simulink model "Tq_comb_timing"  (R2022b)
settings: Solver=daessc  StartTime=0.0  StopTime=5  RelTol=1e-3
InitFcn:
  | %% Tq_comb_timing.slx
  | % InitFcn
  | %
  | spring_stiffness = 1e10;
  | viscous_friction_coeff = 10;
  | current_limit = 12.5;
  | %
  | torque_start_t = 1;
  | torque_fin_val = -45;
  | %
  | inertia_start_t = 11.5;
  | inertia_init_val = 0.1;
  | inertia_fin_val  = 0.2;
  | %
  | M1_start_t = 0;
  | M2_start_t = 2;
  | M3_start_t = 3;
StopFcn:
  | disp(['spring_stiffness was       ' num2str(spring_stiffness)])
  | disp('')
  | disp(['viscous_friction_coeff was ' num2str(viscous_friction_coeff)])
  | disp('')
libraries: fl_lib x73, nesl_utility x42, ee_lib x12, sdl_lib x12, slpidlib x3, SignalEditorBlockLib x1
(part 2 of 2)

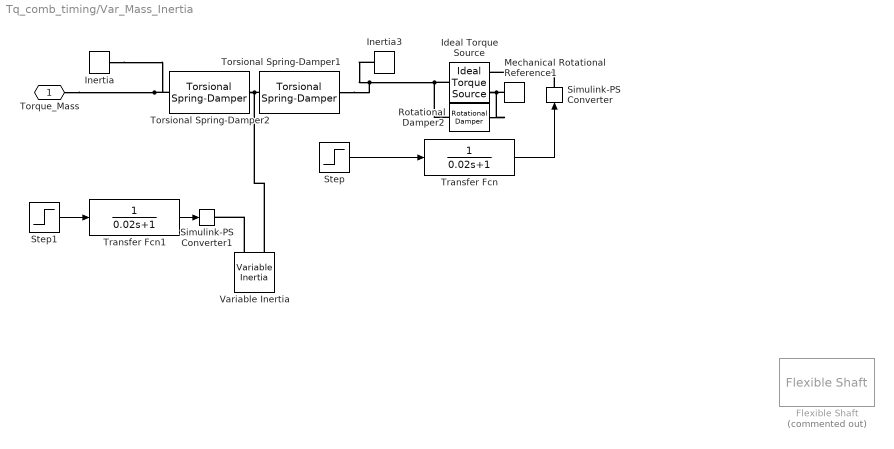
== system Tq_comb_timing/Var_Mass_Inertia ==
  Flexible Shaft : sdl_lib/Couplings & Drives/Flexible Shaft  Commented=on  modelTransverse=simscape.enum.onoff.off  n_segments=1  parameterization=sdl.enum.shaftParameterization.StiffnessInertia  length=1 m  lengths=[1, .5, .25] m  shaft_stiffness=2e5 N*m/rad  shaft_inertia=0.001 kg*m^2  shaft_stiffnesses=[400000, 200000, 100000] N*m/rad  shaft_inertias=[.025, .02, .015] kg*m^2  eiIN=5e5 Pa*m^4  rhoaIN=19 kg/m  eiINs=[600000, 500000, 400000] Pa*m^4  rhoaINs=[20, 19, 18] kg/m  density=7.8e3 kg/m^3  shear_modulus=7.93e9 Pa  elastic_modulus=200e9 Pa  shaft_construction=sdl.enum.shaftConstruction.solid  diameter_outer=0.075 m  diameter_inner=0.05 m  diameter_outers=[.085, .075, .065] m  diameter_inners=[.055, .05, .045] m  damping_ratio=0.01  mu_visc_BF=[0, 0] N*m*s/rad  mu_visc=[0, 0] N*m*s/rad  initial_deflection=0 rad  initial_velocity=0 rpm  num_supports=sdl.enum.num_supports.two  z_support=[0, 1] m  boundaryB1=sdl.enum.shaftSupport.clamp  DrotB1_row=[1000, 1000] N*m*s/rad  DtransB1_row=[20000, -44000, -44000, 350000] N*s/m  DtransB1_w_mat=[20000, -44000, -44000, 350000; 10000, -25000, -25000, 140000; 5000, -10000, -10000, 20000] N*s/m  KrotB1_row=[10000, 10000] N*m/rad  KtransB1_row=[1000000, -200000, -300000, 5000000] N/m  KtransB1_w_mat=[1000000, -600000, -3500000, 8000000; 1000000, -200000, -3000000, 5000000; 1000000, -50000, -2500000, 3000000] N/m  boundaryI1=sdl.enum.shaftSupport.clamp  DrotI1_row=[1000, 1000] N*m*s/rad  DtransI1_row=[20000, -44000, -44000, 350000] N*s/m  DtransI1_w_mat=[20000, -44000, -44000, 350000; 10000, -25000, -25000, 140000; 5000, -10000, -10000, 20000] N*s/m  KrotI1_row=[10000, 10000] N*m/rad  KtransI1_row=[1000000, -200000, -300000, 5000000] N/m  KtransI1_w_mat=[1000000, -600000, -3500000, 8000000; 1000000, -200000, -3000000, 5000000; 1000000, -50000, -2500000, 3000000] N/m  boundaryI2=sdl.enum.shaftSupport.clamp  DrotI2_row=[1000, 1000] N*m*s/rad  DtransI2_row=[20000, -44000, -44000, 350000] N*s/m  DtransI2_w_mat=[20000, -44000, -44000, 350000; 10000, -25000, -25000, 140000; 5000, -10000, -10000, 20000] N*s/m  KrotI2_row=[10000, 10000] N*m/rad  KtransI2_row=[1000000, -200000, -300000, 5000000] N/m  KtransI2_w_mat=[1000000, -600000, -3500000, 8000000; 1000000, -200000, -3000000, 5000000; 1000000, -50000, -2500000, 3000000] N/m  boundaryF1=sdl.enum.shaftSupport.clamp  DrotF1_row=[1000, 1000] N*m*s/rad  DtransF1_row=[20000, -44000, -44000, 350000] N*s/m  DtransF1_w_mat=[20000, -44000, -44000, 350000; 10000, -25000, -25000, 140000; 5000, -10000, -10000, 20000] N*s/m  KrotF1_row=[10000, 10000] N*m/rad  KtransF1_row=[1000000, -200000, -300000, 5000000] N/m  KtransF1_w_mat=[1000000, -600000, -3500000, 8000000; 1000000, -200000, -3000000, 5000000; 1000000, -50000, -2500000, 3000000] N/m  bearing_speed=[200, 500, 1500] rpm  alpha=10 1/s  beta=1e-8 s  noDisk=sdl.enum.shaftDisks.none  zDisk=0.5 m  mDiskIN=2 kg  IdDiskIN=0.025 kg*m^2  IpDiskIN=0.050 kg*m^2  offsetMR=[.01, .01] kg*m  offsetMassLocation=[.33, .67] m  offsetMR_initialAngleIN=[0, pi] rad  AnalysisMethod=sdl.enum.bendingAnalysisMethod.LumpedMass  ModeInputMethod=sdl.enum.modeInputMethod.SimscapeDetermined  numModesIn=6  mode_speed_dependency=sdl.enum.mode_speed_dependency.Static  OmegaNom=5000 rpm  wMax=1e8 rpm  dz=0.01 m  userMode_w=[280, 644, 615, 1285] rad/s  userMode_w_mat=[257, 780, 580, 1560; 280, 644, 615, 1285; 294, 513, 636, 1020] rad/s  userMode_z=[0, .1, .2, .3, .4, .5, .6, .7, .8, .9, 1] m  userMode_shapeX=[.1648, .0086, -.2759, .0162; .1671, .0093, -.2231, .0133; .1691, .01, -.1689, .0102; .1707, .0105, -.1135, .007; .1717, .0108, -.057, .0035; .1721, .0109, 0, 0; .1717, .0108, .057, -.0035; .1707, .0105, .1135, -.007; .1691, .01, .1689, -.0102; .1671, .0093, .2231, -.0133; .1648, .0086, .2759, -.0162]  userMode_shapeX_mat=cat(3, [.1842, .0134, -.3072, .0272; .1863, .0152, -.2482, .0226; .1882, .0169, -.1878, .0176; .1897, .0182, -.1261, .0121; .1906, .019, -.0634, .0062; .191, .0193, 0, 0; .1906, .019, .0634, -.0062; .1897, .0182, .1261, -.0121; .1882, .0169, .1878, -.0176; .1863, .0152, .2482, -.0226; .1842, .0134, .3072, -.0272], [.1648, .0086, -.2759, .0162; .1671, .0093, -.2231, .0133; .1691, .01, -.1689, .0102; .1707, .0105, -.1135, .007; .1717, .0108, -.057, .0035; .1721, .0109, 0, 0; .1717, .0108, .057, -.0035; .1707, .0105, .1135, -.007; .1691, .01, .1689, -.0102; .1671, .0093, .2231, -.0133; .1648, .0086, .2759, -.0162], [.1291, .0046, -.2166, .0082; .131, .0048, -.1751, .0067; .1327, .005, -.1327, .0051; .1341, .0052, -.0891, .0035; .135, .0053, -.0448, .0017; .1353, .0053, 0, 0; .135, .0053, .0448, -.0017; .1341, .0052, .0891, -.0035; .1327, .005, .1327, -.0051; .131, .0048, .1751, -.0067; .1291, .0046, .2166, -.0082])  userMode_shapeY=[.1193, -.1784, -.1997, -.3348; .1209, -.1933, -.1615, -.2751; .1224, -.2068, -.1223, -.2119; .1235, -.2176, -.0821, -.1445; .1243, -.2245, -.0413, -.0734; .1246, -.2269, 0, 0; .1243, -.2245, .0413, .0734; .1235, -.2176, .0821, .1445; .1224, -.2068, .1223, .2119; .1209, -.1933, .1615, .2751; .1193, -.1784, .1997, .3348]  userMode_shapeY_mat=cat(3, [.0885, -.1625, -.1475, -.3301; .0895, -.1847, -.1192, -.2745; .0904, -.2048, -.0902, -.2141; .0911, -.2209, -.0606, -.1475; .0916, -.2313, -.0304, -.0754; .0917, -.2349, 0, 0; .0916, -.2313, .0304, .0754; .0911, -.2209, .0606, .1475; .0904, -.2048, .0902, .2141; .0895, -.1847, .1192, .2745; .0885, -.1625, .1475, .3301], [.1193, -.1784, -.1997, -.3348; .1209, -.1933, -.1615, -.2751; .1224, -.2068, -.1223, -.2119; .1235, -.2176, -.0821, -.1445; .1243, -.2245, -.0413, -.0734; .1246, -.2269, 0, 0; .1243, -.2245, .0413, .0734; .1235, -.2176, .0821, .1445; .1224, -.2068, .1223, .2119; .1209, -.1933, .1615, .2751; .1193, -.1784, .1997, .3348], [.1566, -.1901, -.2628, -.3377; .1589, -.1994, -.2125, -.2753; .161, -.2079, -.1609, -.2103; .1627, -.2146, -.1081, -.1424; .1638, -.219, -.0544, -.0719; .1642, -.2205, 0, 0; .1638, -.219, .0544, .0719; .1627, -.2146, .1081, .1424; .161, -.2079, .1609, .2103; .1589, -.1994, .2125, .2753; .1566, -.1901, .2628, .3377])
      settings: InternalSimscapePortConfiguration="{\"Bottom\":[],\"Left\":[{\"id\":\"B\",\"label\":\"B\",\"type\":\"foundation.mechanical.rotational.rotational\"}],\"Right\":[{\"id\":\"F\",\"label\":\"F\",\"type\":\"foundation.mechanical.rotational.rotational\"}],\"Top\":[]}"
  Ideal Torque Source : fl_lib/Mechanical/Mechanical Sources/Ideal Torque Source
  Inertia : fl_lib/Mechanical/Rotational Elements/Inertia  inertia=0.00001 kg*m^2  num_ports=foundation.enum.numPorts2.one  w_specify=off  w_priority=High  w=0 rad/s  w_nominal_specify=off  w_nominal_unit=rad/s  w_nominal_value=1  t_specify=off  t_priority=None  t=0 N*m  t_nominal_specify=off  t_nominal_unit=N*m  t_nominal_value=1
  Inertia3 : fl_lib/Mechanical/Rotational Elements/Inertia  inertia=0.00001 kg*m^2  num_ports=foundation.enum.numPorts2.one  w_specify=off  w_priority=High  w=0 rad/s  w_nominal_specify=off  w_nominal_unit=rad/s  w_nominal_value=1  t_specify=off  t_priority=None  t=0 N*m  t_nominal_specify=off  t_nominal_unit=N*m  t_nominal_value=1
  Mechanical Rotational Reference1 : fl_lib/Mechanical/Rotational Elements/Mechanical Rotational Reference
  Rotational Damper2 : fl_lib/Mechanical/Rotational Elements/Rotational Damper  D=0.001 N*m*s/rad  w_specify=off  w_priority=None  w=0 rad/s  w_nominal_specify=off  w_nominal_unit=rad/s  w_nominal_value=1  t_specify=off  t_priority=None  t=0 N*m  t_nominal_specify=off  t_nominal_unit=N*m  t_nominal_value=1
  Simulink-PS Converter : nesl_utility/Simulink-PS Converter  PhysicalDomain=network_engine_domain  SubClassName=ps_input  LeftPortType=input  RightPortType=output  PseudoPeriodic=off  Frequencies=[]  NoiseDistribution=none  NoiseParameters=[]  Unit=N*m  AffineConversion=off  FilteringAndDerivatives=provide  SimscapeFilterOrder=1  InputFilterTimeConstant=0.001  UdotUserProvided=0
  Simulink-PS Converter1 : nesl_utility/Simulink-PS Converter  PhysicalDomain=network_engine_domain  SubClassName=ps_input  LeftPortType=input  RightPortType=output  PseudoPeriodic=off  Frequencies=[]  NoiseDistribution=none  NoiseParameters=[]  Unit=kg*m^2  AffineConversion=off  FilteringAndDerivatives=provide  SimscapeFilterOrder=1  InputFilterTimeConstant=0.001  UdotUserProvided=0
  Step : Step  After=-25  SampleTime=0
  Step1 : Step  Time=2  Before=0.1  After=0.5  SampleTime=0
  Torsional Spring-Damper1 : sdl_lib/Couplings & Drives/Torsional Spring-Damper  k=1e7 N*m/rad  mu_visc=1 N*m*s/rad  trq_coulomb=0 N*m  static_kinetic_ratio=1.1  w_tol=0.001 rad/s  model_hardstop=sdl.enum.hardStopOffOn.off  upper_bound=10 deg  lower_bound=-10 deg  k_endstop=1e6 N*m/rad  D_endstop=10 N*m*s/rad  hardstop_model=simscape.enum.hardstop.smooth  transition=0.001 rad  x0=0 deg
      settings: InternalSimscapePortConfiguration="{\"Bottom\":[],\"Left\":[{\"id\":\"R\",\"label\":\"R\",\"type\":\"foundation.mechanical.rotational.rotational\"}],\"Right\":[{\"id\":\"C\",\"label\":\"C\",\"type\":\"foundation.mechanical.rotational.rotational\"}],\"Top\":[]}"
  Torsional Spring-Damper2 : sdl_lib/Couplings & Drives/Torsional Spring-Damper  k=1e7 N*m/rad  mu_visc=1 N*m*s/rad  trq_coulomb=0 N*m  static_kinetic_ratio=1.1  w_tol=0.001 rad/s  model_hardstop=sdl.enum.hardStopOffOn.off  upper_bound=10 deg  lower_bound=-10 deg  k_endstop=1e6 N*m/rad  D_endstop=10 N*m*s/rad  hardstop_model=simscape.enum.hardstop.smooth  transition=0.001 rad  x0=0 deg
      settings: InternalSimscapePortConfiguration="{\"Bottom\":[],\"Left\":[{\"id\":\"R\",\"label\":\"R\",\"type\":\"foundation.mechanical.rotational.rotational\"}],\"Right\":[{\"id\":\"C\",\"label\":\"C\",\"type\":\"foundation.mechanical.rotational.rotational\"}],\"Top\":[]}"
  Transfer Fcn : TransferFcn  Denominator=[0.02 1]
  Transfer Fcn1 : TransferFcn  Denominator=[0.02 1]
  Variable Inertia : sdl_lib/Inertias & Loads/Variable Inertia  minimum_inertia=0.01 kg*m^2  L_specify=on  L_priority=Low  L=0 kg*m^2/s  L_nominal_specify=off  L_nominal_unit=kg*m^2/s  L_nominal_value=1
      settings: InternalSimscapePortConfiguration="{\"Bottom\":[],\"Left\":[{\"id\":\"I\",\"label\":\"\",\"type\":\"input\"},{\"id\":\"A\",\"label\":\"\",\"type\":\"foundation.mechanical.rotational.rotational\"}],\"Right\":[],\"Top\":[]}"
  Torque_Mass : PMIOPort  Side=Right
  wires:
  Step/1 -> Transfer Fcn/1
  Step1/1 -> Transfer Fcn1/1
  Transfer Fcn/1 -> Simulink-PS Converter/1
  Transfer Fcn1/1 -> Simulink-PS Converter1/1
  connections:
  Mechanical Rotational Reference1/LConn1 -- Rotational Damper2/RConn1 -- Ideal Torque Source/RConn2
  Inertia3/LConn1 -- Torsional Spring-Damper1/RConn1 -- Rotational Damper2/LConn1 -- Ideal Torque Source/LConn1
  Torque_Mass/RConn1 -- Inertia/LConn1 -- Torsional Spring-Damper2/LConn1
  Variable Inertia/LConn1 -- Simulink-PS Converter1/RConn1
  Simulink-PS Converter/RConn1 -- Ideal Torque Source/RConn1
  Torsional Spring-Damper1/LConn1 -- Variable Inertia/LConn2 -- Torsional Spring-Damper2/RConn1

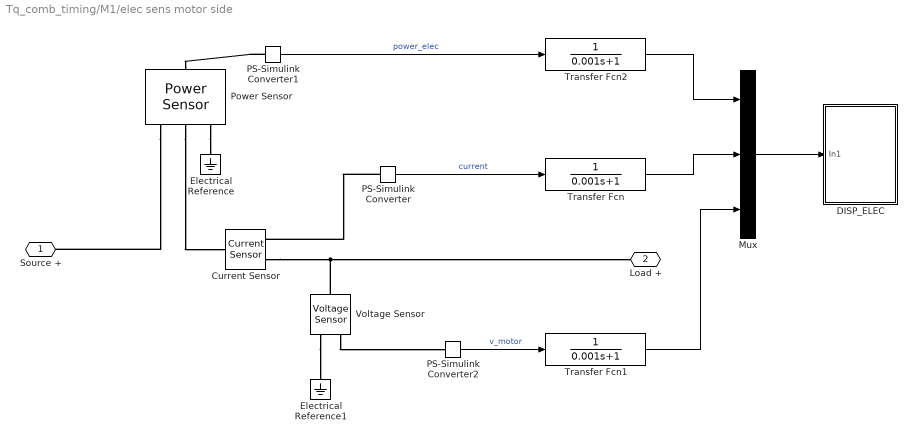
== system Tq_comb_timing/M1/elec sens motor side ==
  Current Sensor : fl_lib/Electrical/Electrical Sensors/Current Sensor
  DISP_ELEC : Subsystem
  Electrical Reference : fl_lib/Electrical/Electrical Elements/Electrical Reference
  Electrical Reference1 : fl_lib/Electrical/Electrical Elements/Electrical Reference
  Mux : Mux  Inputs=3
  PS-Simulink Converter : nesl_utility/PS-Simulink Converter  PhysicalDomain=network_engine_domain  SubClassName=ps_output  LeftPortType=input  RightPortType=output  PseudoPeriodic=off  Frequencies=[]  VectorFormat=inherit  Unit=A  AffineConversion=off
  PS-Simulink Converter1 : nesl_utility/PS-Simulink Converter  PhysicalDomain=network_engine_domain  SubClassName=ps_output  LeftPortType=input  RightPortType=output  PseudoPeriodic=off  Frequencies=[]  VectorFormat=inherit  Unit=W  AffineConversion=off
  PS-Simulink Converter2 : nesl_utility/PS-Simulink Converter  PhysicalDomain=network_engine_domain  SubClassName=ps_output  LeftPortType=input  RightPortType=output  PseudoPeriodic=off  Frequencies=[]  VectorFormat=inherit  Unit=V  AffineConversion=off
  Power Sensor : ee_lib/Sensors & Transducers/Power Sensor  measurement_type=1  averaging_period=1e-4 s
  Transfer Fcn : TransferFcn  Denominator=[0.001 1]
  Transfer Fcn1 : TransferFcn  Denominator=[0.001 1]
  Transfer Fcn2 : TransferFcn  Denominator=[0.001 1]
  Voltage Sensor : fl_lib/Electrical/Electrical Sensors/Voltage Sensor
  Source + : PMIOPort  Side=Left
  Load + : PMIOPort  Port=2  Side=Right
  wires:
  PS-Simulink Converter/1 -> Transfer Fcn/1  "current"
  PS-Simulink Converter1/1 -> Transfer Fcn2/1  "power_elec"
  PS-Simulink Converter2/1 -> Transfer Fcn1/1  "v_motor"
  Transfer Fcn2/1 -> Mux/1
  Transfer Fcn/1 -> Mux/2
  Transfer Fcn1/1 -> Mux/3
  Mux/1 -> DISP_ELEC/1(In1)
  connections:
  Power Sensor/LConn1 -- Source +/RConn1
  Current Sensor/RConn2 -- Load +/RConn1 -- Voltage Sensor/LConn1
  PS-Simulink Converter/LConn1 -- Current Sensor/RConn1
  PS-Simulink Converter1/LConn1 -- Power Sensor/RConn1
  Voltage Sensor/RConn2 -- Electrical Reference1/LConn1
  Voltage Sensor/RConn1 -- PS-Simulink Converter2/LConn1
  Power Sensor/LConn2 -- Current Sensor/LConn1
  Power Sensor/LConn3 -- Electrical Reference/LConn1

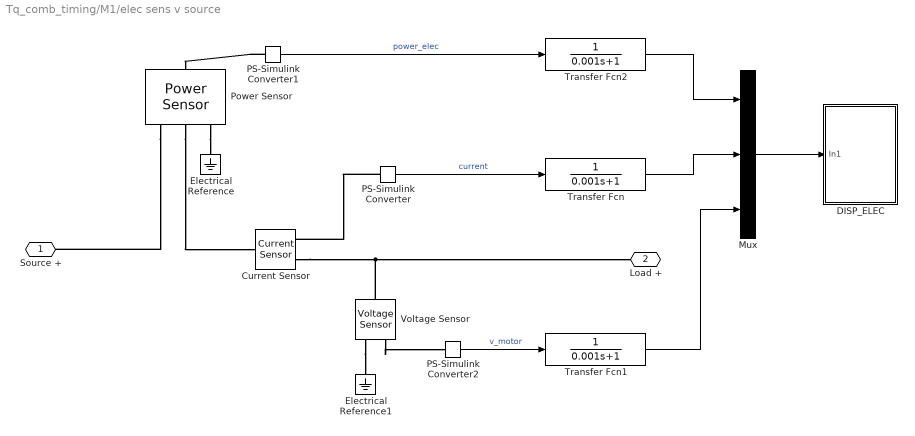
== system Tq_comb_timing/M1/elec sens v source ==
  Current Sensor : fl_lib/Electrical/Electrical Sensors/Current Sensor
  DISP_ELEC : Subsystem
  Electrical Reference : fl_lib/Electrical/Electrical Elements/Electrical Reference
  Electrical Reference1 : fl_lib/Electrical/Electrical Elements/Electrical Reference
  Mux : Mux  Inputs=3
  PS-Simulink Converter : nesl_utility/PS-Simulink Converter  PhysicalDomain=network_engine_domain  SubClassName=ps_output  LeftPortType=input  RightPortType=output  PseudoPeriodic=off  Frequencies=[]  VectorFormat=inherit  Unit=A  AffineConversion=off
  PS-Simulink Converter1 : nesl_utility/PS-Simulink Converter  PhysicalDomain=network_engine_domain  SubClassName=ps_output  LeftPortType=input  RightPortType=output  PseudoPeriodic=off  Frequencies=[]  VectorFormat=inherit  Unit=W  AffineConversion=off
  PS-Simulink Converter2 : nesl_utility/PS-Simulink Converter  PhysicalDomain=network_engine_domain  SubClassName=ps_output  LeftPortType=input  RightPortType=output  PseudoPeriodic=off  Frequencies=[]  VectorFormat=inherit  Unit=V  AffineConversion=off
  Power Sensor : ee_lib/Sensors & Transducers/Power Sensor  measurement_type=1  averaging_period=1e-4 s
  Transfer Fcn : TransferFcn  Denominator=[0.001 1]
  Transfer Fcn1 : TransferFcn  Denominator=[0.001 1]
  Transfer Fcn2 : TransferFcn  Denominator=[0.001 1]
  Voltage Sensor : fl_lib/Electrical/Electrical Sensors/Voltage Sensor
  Source + : PMIOPort  Side=Left
  Load + : PMIOPort  Port=2  Side=Right
  wires:
  Mux/1 -> DISP_ELEC/1(In1)
  Transfer Fcn1/1 -> Mux/3
  Transfer Fcn/1 -> Mux/2
  Transfer Fcn2/1 -> Mux/1
  PS-Simulink Converter2/1 -> Transfer Fcn1/1  "v_motor"
  PS-Simulink Converter1/1 -> Transfer Fcn2/1  "power_elec"
  PS-Simulink Converter/1 -> Transfer Fcn/1  "current"
  connections:
  Power Sensor/LConn3 -- Electrical Reference/LConn1
  Power Sensor/LConn2 -- Current Sensor/LConn1
  Voltage Sensor/RConn1 -- PS-Simulink Converter2/LConn1
  Voltage Sensor/RConn2 -- Electrical Reference1/LConn1
  PS-Simulink Converter1/LConn1 -- Power Sensor/RConn1
  PS-Simulink Converter/LConn1 -- Current Sensor/RConn1
  Voltage Sensor/LConn1 -- Load +/RConn1 -- Current Sensor/RConn2
  Power Sensor/LConn1 -- Source +/RConn1

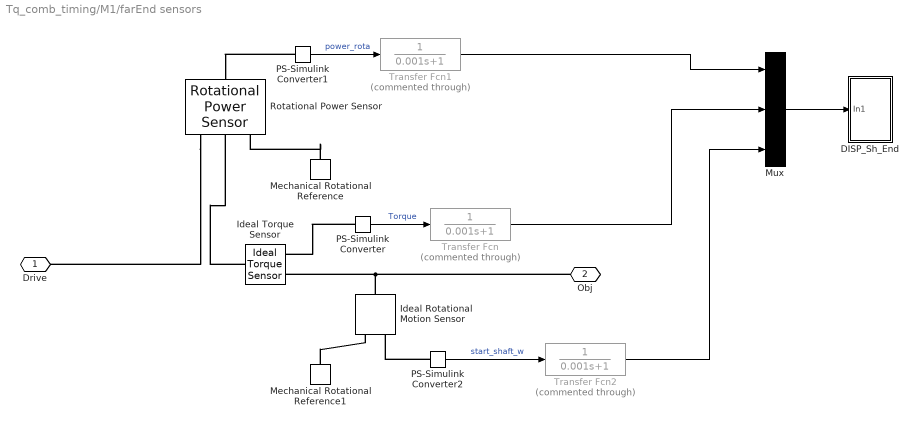
== system Tq_comb_timing/M1/farEnd sensors ==
  DISP_Sh_End : Subsystem
  Ideal Rotational Motion Sensor : fl_lib/Mechanical/Mechanical Sensors/Ideal Rotational Motion Sensor  reference=foundation.enum.MeasurementReference.difference  acceleration_port=false  velocity_port=true  position_port=false  wrap_angle=false  offset=0 rad
      settings: InternalSimscapePortConfiguration="{\"Bottom\":[],\"Left\":[{\"id\":\"R\",\"label\":\"R\",\"type\":\"foundation.mechanical.rotational.rotational\"}],\"Right\":[{\"id\":\"C\",\"label\":\"C\",\"type\":\"foundation.mechanical.rotational.rotational\"},{\"id\":\"W\",\"label\":\"W\",\"type\":\"output\"}],\"Top\":[]}"
  Ideal Torque Sensor : fl_lib/Mechanical/Mechanical Sensors/Ideal Torque Sensor
  Mechanical Rotational Reference : fl_lib/Mechanical/Rotational Elements/Mechanical Rotational Reference
  Mechanical Rotational Reference1 : fl_lib/Mechanical/Rotational Elements/Mechanical Rotational Reference
  Mux : Mux  Inputs=3
  PS-Simulink Converter : nesl_utility/PS-Simulink Converter  PhysicalDomain=network_engine_domain  SubClassName=ps_output  LeftPortType=input  RightPortType=output  PseudoPeriodic=off  Frequencies=[]  VectorFormat=inherit  Unit=inherit  AffineConversion=off
  PS-Simulink Converter1 : nesl_utility/PS-Simulink Converter  PhysicalDomain=network_engine_domain  SubClassName=ps_output  LeftPortType=input  RightPortType=output  PseudoPeriodic=off  Frequencies=[]  VectorFormat=inherit  Unit=W  AffineConversion=off
  PS-Simulink Converter2 : nesl_utility/PS-Simulink Converter  PhysicalDomain=network_engine_domain  SubClassName=ps_output  LeftPortType=input  RightPortType=output  PseudoPeriodic=off  Frequencies=[]  VectorFormat=inherit  Unit=rpm  AffineConversion=off
  Rotational Power Sensor : sdl_lib/Sensors/Rotational Power Sensor  measurement_type=sdl.enum.rotationalPowerSensorType.instantaneous  averaging_period=1 s  max_frequency=1000 Hz  max_speed=1000 rpm
      settings: InternalSimscapePortConfiguration="{\"Bottom\":[],\"Left\":[{\"id\":\"S\",\"label\":\"S\",\"type\":\"foundation.mechanical.rotational.rotational\"},{\"id\":\"R\",\"label\":\"R\",\"type\":\"foundation.mechanical.rotational.rotational\"},{\"id\":\"C\",\"label\":\"C\",\"type\":\"foundation.mechanical.rotational.rotational\"}],\"Right\":[{\"id\":\"P\",\"label\":\"P\",\"type\":\"output\"}],\"Top\":[]}"
  Transfer Fcn : TransferFcn  Commented=through  Denominator=[0.001 1]
  Transfer Fcn1 : TransferFcn  Commented=through  Denominator=[0.001 1]
  Transfer Fcn2 : TransferFcn  Commented=through  Denominator=[0.001 1]
  Drive : PMIOPort  Side=Left
  Obj : PMIOPort  Port=2  Side=Right
  wires:
  PS-Simulink Converter/1 -> Transfer Fcn/1  "Torque"
  PS-Simulink Converter1/1 -> Transfer Fcn1/1  "power_rota"
  PS-Simulink Converter2/1 -> Transfer Fcn2/1  "start_shaft_w"
  Transfer Fcn1/1 -> Mux/1
  Transfer Fcn/1 -> Mux/2
  Transfer Fcn2/1 -> Mux/3
  Mux/1 -> DISP_Sh_End/1(In1)
  connections:
  Rotational Power Sensor/LConn1 -- Drive/RConn1
  Obj/RConn1 -- Ideal Rotational Motion Sensor/LConn1 -- Ideal Torque Sensor/RConn1
  PS-Simulink Converter/LConn1 -- Ideal Torque Sensor/RConn2
  Mechanical Rotational Reference/LConn1 -- Rotational Power Sensor/LConn3
  PS-Simulink Converter1/LConn1 -- Rotational Power Sensor/RConn1
  Mechanical Rotational Reference1/LConn1 -- Ideal Rotational Motion Sensor/RConn1
  PS-Simulink Converter2/LConn1 -- Ideal Rotational Motion Sensor/RConn2
  Ideal Torque Sensor/LConn1 -- Rotational Power Sensor/LConn2

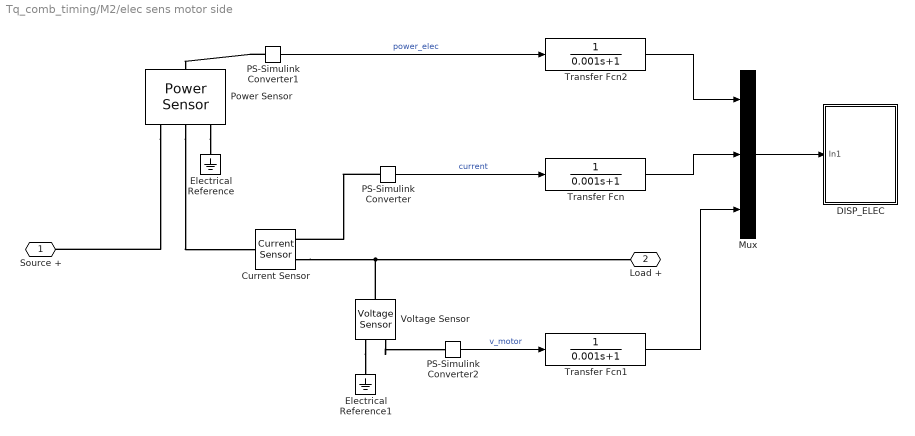
== system Tq_comb_timing/M2/elec sens motor side ==
  Current Sensor : fl_lib/Electrical/Electrical Sensors/Current Sensor
  DISP_ELEC : Subsystem
  Electrical Reference : fl_lib/Electrical/Electrical Elements/Electrical Reference
  Electrical Reference1 : fl_lib/Electrical/Electrical Elements/Electrical Reference
  Mux : Mux  Inputs=3
  PS-Simulink Converter : nesl_utility/PS-Simulink Converter  PhysicalDomain=network_engine_domain  SubClassName=ps_output  LeftPortType=input  RightPortType=output  PseudoPeriodic=off  Frequencies=[]  VectorFormat=inherit  Unit=A  AffineConversion=off
  PS-Simulink Converter1 : nesl_utility/PS-Simulink Converter  PhysicalDomain=network_engine_domain  SubClassName=ps_output  LeftPortType=input  RightPortType=output  PseudoPeriodic=off  Frequencies=[]  VectorFormat=inherit  Unit=W  AffineConversion=off
  PS-Simulink Converter2 : nesl_utility/PS-Simulink Converter  PhysicalDomain=network_engine_domain  SubClassName=ps_output  LeftPortType=input  RightPortType=output  PseudoPeriodic=off  Frequencies=[]  VectorFormat=inherit  Unit=V  AffineConversion=off
  Power Sensor : ee_lib/Sensors & Transducers/Power Sensor  measurement_type=1  averaging_period=1e-4 s
  Transfer Fcn : TransferFcn  Denominator=[0.001 1]
  Transfer Fcn1 : TransferFcn  Denominator=[0.001 1]
  Transfer Fcn2 : TransferFcn  Denominator=[0.001 1]
  Voltage Sensor : fl_lib/Electrical/Electrical Sensors/Voltage Sensor
  Source + : PMIOPort  Side=Left
  Load + : PMIOPort  Port=2  Side=Right
  wires:
  Mux/1 -> DISP_ELEC/1(In1)
  Transfer Fcn1/1 -> Mux/3
  Transfer Fcn/1 -> Mux/2
  Transfer Fcn2/1 -> Mux/1
  PS-Simulink Converter2/1 -> Transfer Fcn1/1  "v_motor"
  PS-Simulink Converter1/1 -> Transfer Fcn2/1  "power_elec"
  PS-Simulink Converter/1 -> Transfer Fcn/1  "current"
  connections:
  Power Sensor/LConn3 -- Electrical Reference/LConn1
  Power Sensor/LConn2 -- Current Sensor/LConn1
  Voltage Sensor/RConn1 -- PS-Simulink Converter2/LConn1
  Voltage Sensor/RConn2 -- Electrical Reference1/LConn1
  PS-Simulink Converter1/LConn1 -- Power Sensor/RConn1
  PS-Simulink Converter/LConn1 -- Current Sensor/RConn1
  Voltage Sensor/LConn1 -- Load +/RConn1 -- Current Sensor/RConn2
  Power Sensor/LConn1 -- Source +/RConn1

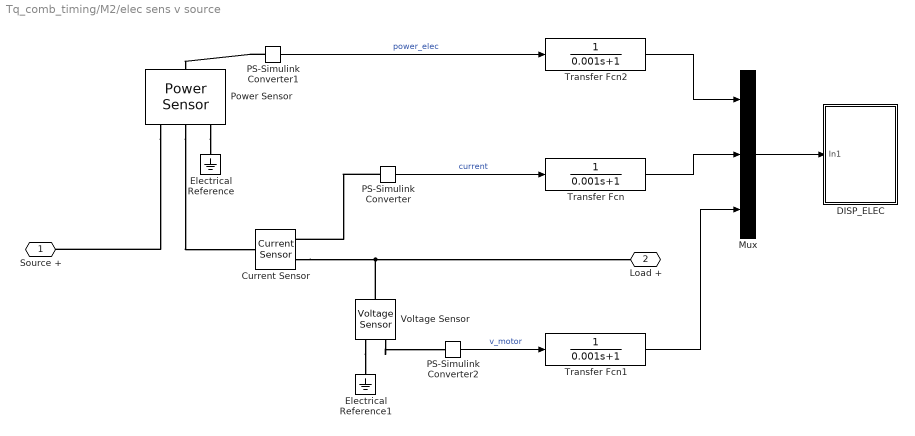
== system Tq_comb_timing/M2/elec sens v source ==
  Current Sensor : fl_lib/Electrical/Electrical Sensors/Current Sensor
  DISP_ELEC : Subsystem
  Electrical Reference : fl_lib/Electrical/Electrical Elements/Electrical Reference
  Electrical Reference1 : fl_lib/Electrical/Electrical Elements/Electrical Reference
  Mux : Mux  Inputs=3
  PS-Simulink Converter : nesl_utility/PS-Simulink Converter  PhysicalDomain=network_engine_domain  SubClassName=ps_output  LeftPortType=input  RightPortType=output  PseudoPeriodic=off  Frequencies=[]  VectorFormat=inherit  Unit=A  AffineConversion=off
  PS-Simulink Converter1 : nesl_utility/PS-Simulink Converter  PhysicalDomain=network_engine_domain  SubClassName=ps_output  LeftPortType=input  RightPortType=output  PseudoPeriodic=off  Frequencies=[]  VectorFormat=inherit  Unit=W  AffineConversion=off
  PS-Simulink Converter2 : nesl_utility/PS-Simulink Converter  PhysicalDomain=network_engine_domain  SubClassName=ps_output  LeftPortType=input  RightPortType=output  PseudoPeriodic=off  Frequencies=[]  VectorFormat=inherit  Unit=V  AffineConversion=off
  Power Sensor : ee_lib/Sensors & Transducers/Power Sensor  measurement_type=1  averaging_period=1e-4 s
  Transfer Fcn : TransferFcn  Denominator=[0.001 1]
  Transfer Fcn1 : TransferFcn  Denominator=[0.001 1]
  Transfer Fcn2 : TransferFcn  Denominator=[0.001 1]
  Voltage Sensor : fl_lib/Electrical/Electrical Sensors/Voltage Sensor
  Source + : PMIOPort  Side=Left
  Load + : PMIOPort  Port=2  Side=Right
  wires:
  PS-Simulink Converter/1 -> Transfer Fcn/1  "current"
  PS-Simulink Converter1/1 -> Transfer Fcn2/1  "power_elec"
  PS-Simulink Converter2/1 -> Transfer Fcn1/1  "v_motor"
  Transfer Fcn2/1 -> Mux/1
  Transfer Fcn/1 -> Mux/2
  Transfer Fcn1/1 -> Mux/3
  Mux/1 -> DISP_ELEC/1(In1)
  connections:
  Power Sensor/LConn1 -- Source +/RConn1
  Current Sensor/RConn2 -- Load +/RConn1 -- Voltage Sensor/LConn1
  PS-Simulink Converter/LConn1 -- Current Sensor/RConn1
  PS-Simulink Converter1/LConn1 -- Power Sensor/RConn1
  Voltage Sensor/RConn2 -- Electrical Reference1/LConn1
  Voltage Sensor/RConn1 -- PS-Simulink Converter2/LConn1
  Power Sensor/LConn2 -- Current Sensor/LConn1
  Power Sensor/LConn3 -- Electrical Reference/LConn1

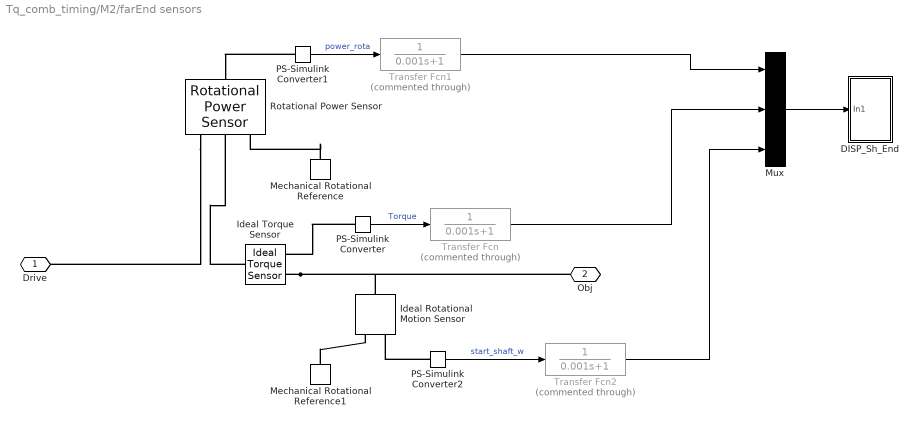
== system Tq_comb_timing/M2/farEnd sensors ==
  DISP_Sh_End : Subsystem
  Ideal Rotational Motion Sensor : fl_lib/Mechanical/Mechanical Sensors/Ideal Rotational Motion Sensor  reference=foundation.enum.MeasurementReference.difference  acceleration_port=false  velocity_port=true  position_port=false  wrap_angle=false  offset=0 rad
      settings: InternalSimscapePortConfiguration="{\"Bottom\":[],\"Left\":[{\"id\":\"R\",\"label\":\"R\",\"type\":\"foundation.mechanical.rotational.rotational\"}],\"Right\":[{\"id\":\"C\",\"label\":\"C\",\"type\":\"foundation.mechanical.rotational.rotational\"},{\"id\":\"W\",\"label\":\"W\",\"type\":\"output\"}],\"Top\":[]}"
  Ideal Torque Sensor : fl_lib/Mechanical/Mechanical Sensors/Ideal Torque Sensor
  Mechanical Rotational Reference : fl_lib/Mechanical/Rotational Elements/Mechanical Rotational Reference
  Mechanical Rotational Reference1 : fl_lib/Mechanical/Rotational Elements/Mechanical Rotational Reference
  Mux : Mux  Inputs=3
  PS-Simulink Converter : nesl_utility/PS-Simulink Converter  PhysicalDomain=network_engine_domain  SubClassName=ps_output  LeftPortType=input  RightPortType=output  PseudoPeriodic=off  Frequencies=[]  VectorFormat=inherit  Unit=inherit  AffineConversion=off
  PS-Simulink Converter1 : nesl_utility/PS-Simulink Converter  PhysicalDomain=network_engine_domain  SubClassName=ps_output  LeftPortType=input  RightPortType=output  PseudoPeriodic=off  Frequencies=[]  VectorFormat=inherit  Unit=W  AffineConversion=off
  PS-Simulink Converter2 : nesl_utility/PS-Simulink Converter  PhysicalDomain=network_engine_domain  SubClassName=ps_output  LeftPortType=input  RightPortType=output  PseudoPeriodic=off  Frequencies=[]  VectorFormat=inherit  Unit=rpm  AffineConversion=off
  Rotational Power Sensor : sdl_lib/Sensors/Rotational Power Sensor  measurement_type=sdl.enum.rotationalPowerSensorType.instantaneous  averaging_period=1 s  max_frequency=1000 Hz  max_speed=1000 rpm
      settings: InternalSimscapePortConfiguration="{\"Bottom\":[],\"Left\":[{\"id\":\"S\",\"label\":\"S\",\"type\":\"foundation.mechanical.rotational.rotational\"},{\"id\":\"R\",\"label\":\"R\",\"type\":\"foundation.mechanical.rotational.rotational\"},{\"id\":\"C\",\"label\":\"C\",\"type\":\"foundation.mechanical.rotational.rotational\"}],\"Right\":[{\"id\":\"P\",\"label\":\"P\",\"type\":\"output\"}],\"Top\":[]}"
  Transfer Fcn : TransferFcn  Commented=through  Denominator=[0.001 1]
  Transfer Fcn1 : TransferFcn  Commented=through  Denominator=[0.001 1]
  Transfer Fcn2 : TransferFcn  Commented=through  Denominator=[0.001 1]
  Drive : PMIOPort  Side=Left
  Obj : PMIOPort  Port=2  Side=Right
  wires:
  Mux/1 -> DISP_Sh_End/1(In1)
  Transfer Fcn2/1 -> Mux/3
  Transfer Fcn/1 -> Mux/2
  Transfer Fcn1/1 -> Mux/1
  PS-Simulink Converter2/1 -> Transfer Fcn2/1  "start_shaft_w"
  PS-Simulink Converter1/1 -> Transfer Fcn1/1  "power_rota"
  PS-Simulink Converter/1 -> Transfer Fcn/1  "Torque"
  connections:
  Ideal Torque Sensor/LConn1 -- Rotational Power Sensor/LConn2
  PS-Simulink Converter2/LConn1 -- Ideal Rotational Motion Sensor/RConn2
  Mechanical Rotational Reference1/LConn1 -- Ideal Rotational Motion Sensor/RConn1
  PS-Simulink Converter1/LConn1 -- Rotational Power Sensor/RConn1
  Mechanical Rotational Reference/LConn1 -- Rotational Power Sensor/LConn3
  PS-Simulink Converter/LConn1 -- Ideal Torque Sensor/RConn2
  Ideal Torque Sensor/RConn1 -- Ideal Rotational Motion Sensor/LConn1 -- Obj/RConn1
  Rotational Power Sensor/LConn1 -- Drive/RConn1

== system Tq_comb_timing/M3/elec sens motor side ==
  Current Sensor : fl_lib/Electrical/Electrical Sensors/Current Sensor
  DISP_ELEC : Subsystem
  Electrical Reference : fl_lib/Electrical/Electrical Elements/Electrical Reference
  Electrical Reference1 : fl_lib/Electrical/Electrical Elements/Electrical Reference
  Mux : Mux  Inputs=3
  PS-Simulink Converter : nesl_utility/PS-Simulink Converter  PhysicalDomain=network_engine_domain  SubClassName=ps_output  LeftPortType=input  RightPortType=output  PseudoPeriodic=off  Frequencies=[]  VectorFormat=inherit  Unit=A  AffineConversion=off
  PS-Simulink Converter1 : nesl_utility/PS-Simulink Converter  PhysicalDomain=network_engine_domain  SubClassName=ps_output  LeftPortType=input  RightPortType=output  PseudoPeriodic=off  Frequencies=[]  VectorFormat=inherit  Unit=W  AffineConversion=off
  PS-Simulink Converter2 : nesl_utility/PS-Simulink Converter  PhysicalDomain=network_engine_domain  SubClassName=ps_output  LeftPortType=input  RightPortType=output  PseudoPeriodic=off  Frequencies=[]  VectorFormat=inherit  Unit=V  AffineConversion=off
  Power Sensor : ee_lib/Sensors & Transducers/Power Sensor  measurement_type=1  averaging_period=1e-4 s
  Transfer Fcn : TransferFcn  Denominator=[0.001 1]
  Transfer Fcn1 : TransferFcn  Denominator=[0.001 1]
  Transfer Fcn2 : TransferFcn  Denominator=[0.001 1]
  Voltage Sensor : fl_lib/Electrical/Electrical Sensors/Voltage Sensor
  Source + : PMIOPort  Side=Left
  Load + : PMIOPort  Port=2  Side=Right
  wires:
  PS-Simulink Converter/1 -> Transfer Fcn/1  "current"
  PS-Simulink Converter1/1 -> Transfer Fcn2/1  "power_elec"
  PS-Simulink Converter2/1 -> Transfer Fcn1/1  "v_motor"
  Transfer Fcn2/1 -> Mux/1
  Transfer Fcn/1 -> Mux/2
  Transfer Fcn1/1 -> Mux/3
  Mux/1 -> DISP_ELEC/1(In1)
  connections:
  Power Sensor/LConn1 -- Source +/RConn1
  Current Sensor/RConn2 -- Load +/RConn1 -- Voltage Sensor/LConn1
  PS-Simulink Converter/LConn1 -- Current Sensor/RConn1
  PS-Simulink Converter1/LConn1 -- Power Sensor/RConn1
  Voltage Sensor/RConn2 -- Electrical Reference1/LConn1
  Voltage Sensor/RConn1 -- PS-Simulink Converter2/LConn1
  Power Sensor/LConn2 -- Current Sensor/LConn1
  Power Sensor/LConn3 -- Electrical Reference/LConn1

== system Tq_comb_timing/M3/elec sens v source ==
  Current Sensor : fl_lib/Electrical/Electrical Sensors/Current Sensor
  DISP_ELEC : Subsystem
  Electrical Reference : fl_lib/Electrical/Electrical Elements/Electrical Reference
  Electrical Reference1 : fl_lib/Electrical/Electrical Elements/Electrical Reference
  Mux : Mux  Inputs=3
  PS-Simulink Converter : nesl_utility/PS-Simulink Converter  PhysicalDomain=network_engine_domain  SubClassName=ps_output  LeftPortType=input  RightPortType=output  PseudoPeriodic=off  Frequencies=[]  VectorFormat=inherit  Unit=A  AffineConversion=off
  PS-Simulink Converter1 : nesl_utility/PS-Simulink Converter  PhysicalDomain=network_engine_domain  SubClassName=ps_output  LeftPortType=input  RightPortType=output  PseudoPeriodic=off  Frequencies=[]  VectorFormat=inherit  Unit=W  AffineConversion=off
  PS-Simulink Converter2 : nesl_utility/PS-Simulink Converter  PhysicalDomain=network_engine_domain  SubClassName=ps_output  LeftPortType=input  RightPortType=output  PseudoPeriodic=off  Frequencies=[]  VectorFormat=inherit  Unit=V  AffineConversion=off
  Power Sensor : ee_lib/Sensors & Transducers/Power Sensor  measurement_type=1  averaging_period=1e-4 s
  Transfer Fcn : TransferFcn  Denominator=[0.001 1]
  Transfer Fcn1 : TransferFcn  Denominator=[0.001 1]
  Transfer Fcn2 : TransferFcn  Denominator=[0.001 1]
  Voltage Sensor : fl_lib/Electrical/Electrical Sensors/Voltage Sensor
  Source + : PMIOPort  Side=Left
  Load + : PMIOPort  Port=2  Side=Right
  wires:
  Mux/1 -> DISP_ELEC/1(In1)
  Transfer Fcn1/1 -> Mux/3
  Transfer Fcn/1 -> Mux/2
  Transfer Fcn2/1 -> Mux/1
  PS-Simulink Converter2/1 -> Transfer Fcn1/1  "v_motor"
  PS-Simulink Converter1/1 -> Transfer Fcn2/1  "power_elec"
  PS-Simulink Converter/1 -> Transfer Fcn/1  "current"
  connections:
  Power Sensor/LConn3 -- Electrical Reference/LConn1
  Power Sensor/LConn2 -- Current Sensor/LConn1
  Voltage Sensor/RConn1 -- PS-Simulink Converter2/LConn1
  Voltage Sensor/RConn2 -- Electrical Reference1/LConn1
  PS-Simulink Converter1/LConn1 -- Power Sensor/RConn1
  PS-Simulink Converter/LConn1 -- Current Sensor/RConn1
  Voltage Sensor/LConn1 -- Load +/RConn1 -- Current Sensor/RConn2
  Power Sensor/LConn1 -- Source +/RConn1

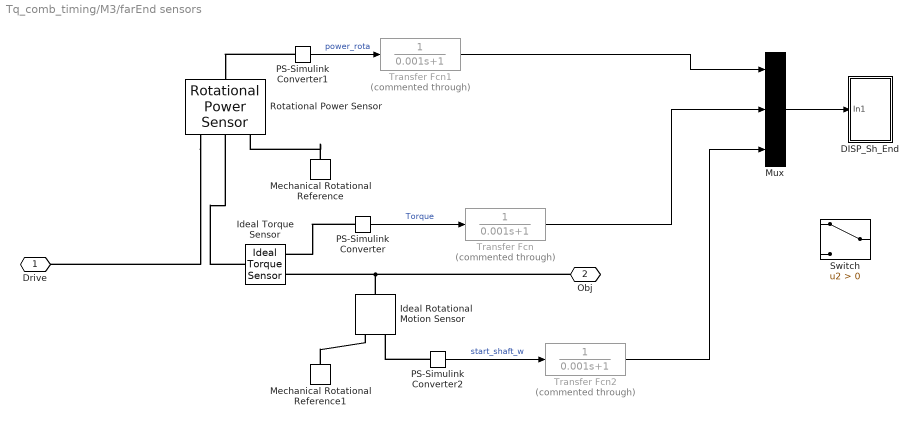
== system Tq_comb_timing/M3/farEnd sensors ==
  DISP_Sh_End : Subsystem
  Ideal Rotational Motion Sensor : fl_lib/Mechanical/Mechanical Sensors/Ideal Rotational Motion Sensor  reference=foundation.enum.MeasurementReference.difference  acceleration_port=false  velocity_port=true  position_port=false  wrap_angle=false  offset=0 rad
      settings: InternalSimscapePortConfiguration="{\"Bottom\":[],\"Left\":[{\"id\":\"R\",\"label\":\"R\",\"type\":\"foundation.mechanical.rotational.rotational\"}],\"Right\":[{\"id\":\"C\",\"label\":\"C\",\"type\":\"foundation.mechanical.rotational.rotational\"},{\"id\":\"W\",\"label\":\"W\",\"type\":\"output\"}],\"Top\":[]}"
  Ideal Torque Sensor : fl_lib/Mechanical/Mechanical Sensors/Ideal Torque Sensor
  Mechanical Rotational Reference : fl_lib/Mechanical/Rotational Elements/Mechanical Rotational Reference
  Mechanical Rotational Reference1 : fl_lib/Mechanical/Rotational Elements/Mechanical Rotational Reference
  Mux : Mux  Inputs=3
  PS-Simulink Converter : nesl_utility/PS-Simulink Converter  PhysicalDomain=network_engine_domain  SubClassName=ps_output  LeftPortType=input  RightPortType=output  PseudoPeriodic=off  Frequencies=[]  VectorFormat=inherit  Unit=inherit  AffineConversion=off
  PS-Simulink Converter1 : nesl_utility/PS-Simulink Converter  PhysicalDomain=network_engine_domain  SubClassName=ps_output  LeftPortType=input  RightPortType=output  PseudoPeriodic=off  Frequencies=[]  VectorFormat=inherit  Unit=W  AffineConversion=off
  PS-Simulink Converter2 : nesl_utility/PS-Simulink Converter  PhysicalDomain=network_engine_domain  SubClassName=ps_output  LeftPortType=input  RightPortType=output  PseudoPeriodic=off  Frequencies=[]  VectorFormat=inherit  Unit=rpm  AffineConversion=off
  Rotational Power Sensor : sdl_lib/Sensors/Rotational Power Sensor  measurement_type=sdl.enum.rotationalPowerSensorType.instantaneous  averaging_period=1 s  max_frequency=1000 Hz  max_speed=1000 rpm
      settings: InternalSimscapePortConfiguration="{\"Bottom\":[],\"Left\":[{\"id\":\"S\",\"label\":\"S\",\"type\":\"foundation.mechanical.rotational.rotational\"},{\"id\":\"R\",\"label\":\"R\",\"type\":\"foundation.mechanical.rotational.rotational\"},{\"id\":\"C\",\"label\":\"C\",\"type\":\"foundation.mechanical.rotational.rotational\"}],\"Right\":[{\"id\":\"P\",\"label\":\"P\",\"type\":\"output\"}],\"Top\":[]}"
  Switch : Switch  Criteria=u2 > Threshold  SaturateOnIntegerOverflow=off  InputSameDT=off
  Transfer Fcn : TransferFcn  Commented=through  Denominator=[0.001 1]
  Transfer Fcn1 : TransferFcn  Commented=through  Denominator=[0.001 1]
  Transfer Fcn2 : TransferFcn  Commented=through  Denominator=[0.001 1]
  Drive : PMIOPort  Side=Left
  Obj : PMIOPort  Port=2  Side=Right
  wires:
  PS-Simulink Converter/1 -> Transfer Fcn/1  "Torque"
  PS-Simulink Converter1/1 -> Transfer Fcn1/1  "power_rota"
  PS-Simulink Converter2/1 -> Transfer Fcn2/1  "start_shaft_w"
  Transfer Fcn1/1 -> Mux/1
  Transfer Fcn/1 -> Mux/2
  Transfer Fcn2/1 -> Mux/3
  Mux/1 -> DISP_Sh_End/1(In1)
  connections:
  Rotational Power Sensor/LConn1 -- Drive/RConn1
  Obj/RConn1 -- Ideal Rotational Motion Sensor/LConn1 -- Ideal Torque Sensor/RConn1
  PS-Simulink Converter/LConn1 -- Ideal Torque Sensor/RConn2
  Mechanical Rotational Reference/LConn1 -- Rotational Power Sensor/LConn3
  PS-Simulink Converter1/LConn1 -- Rotational Power Sensor/RConn1
  Mechanical Rotational Reference1/LConn1 -- Ideal Rotational Motion Sensor/RConn1
  PS-Simulink Converter2/LConn1 -- Ideal Rotational Motion Sensor/RConn2
  Ideal Torque Sensor/LConn1 -- Rotational Power Sensor/LConn2

== system Tq_comb_timing/M1/elec sens motor side/DISP_ELEC ==
  In1 : Inport
  Demux : Demux  Outputs=3
  tag scope: current_M1=global, power_elec_M1=global, v_motor_M1=global
  wires:
  Demux/2 -> [current_M1]
  Demux/1 -> [power_elec_M1]
  Demux/3 -> [v_motor_M1]
  In1/1 -> Demux/1

== system Tq_comb_timing/M1/elec sens v source/DISP_ELEC ==
  In1 : Inport
  Demux : Demux  Outputs=3
  Terminator : Terminator
  Terminator1 : Terminator
  tag scope: v_in_M1=global
  wires:
  In1/1 -> Demux/1
  Demux/3 -> [v_in_M1]
  Demux/1 -> Terminator1/1
  Demux/2 -> Terminator/1

== system Tq_comb_timing/M1/farEnd sensors/DISP_Sh_End ==
  In1 : Inport
  Demux : Demux  Outputs=3
  tag scope: Speed_M1=global, power_rota_M1=global, torque_M1=global
  wires:
  In1/1 -> Demux/1
  Demux/1 -> [power_rota_M1]
  Demux/2 -> [torque_M1]
  Demux/3 -> [Speed_M1]

== system Tq_comb_timing/M2/elec sens motor side/DISP_ELEC ==
  In1 : Inport
  Demux : Demux  Outputs=3
  tag scope: current_M2=global, power_elec_M2=global, v_motor_M2=global
  wires:
  In1/1 -> Demux/1
  Demux/3 -> [v_motor_M2]
  Demux/1 -> [power_elec_M2]
  Demux/2 -> [current_M2]

== system Tq_comb_timing/M2/elec sens v source/DISP_ELEC ==
  In1 : Inport
  Demux : Demux  Outputs=3
  Terminator : Terminator
  Terminator1 : Terminator
  tag scope: v_in_M2=global
  wires:
  Demux/2 -> Terminator/1
  Demux/1 -> Terminator1/1
  Demux/3 -> [v_in_M2]
  In1/1 -> Demux/1

== system Tq_comb_timing/M2/farEnd sensors/DISP_Sh_End ==
  In1 : Inport
  Demux : Demux  Outputs=3
  tag scope: Speed_M2=global, power_rota_M2=global, torque_M2=global
  wires:
  Demux/3 -> [Speed_M2]
  Demux/2 -> [torque_M2]
  Demux/1 -> [power_rota_M2]
  In1/1 -> Demux/1

== system Tq_comb_timing/M3/elec sens motor side/DISP_ELEC ==
  In1 : Inport
  Demux : Demux  Outputs=3
  tag scope: current_M3=global, power_elec_M3=global, v_motor_M3=global
  wires:
  Demux/2 -> [current_M3]
  Demux/1 -> [power_elec_M3]
  Demux/3 -> [v_motor_M3]
  In1/1 -> Demux/1

== system Tq_comb_timing/M3/elec sens v source/DISP_ELEC ==
  In1 : Inport
  Demux : Demux  Outputs=3
  Terminator : Terminator
  Terminator1 : Terminator
  tag scope: v_in_M3=global
  wires:
  In1/1 -> Demux/1
  Demux/3 -> [v_in_M3]
  Demux/1 -> Terminator1/1
  Demux/2 -> Terminator/1

== system Tq_comb_timing/M3/farEnd sensors/DISP_Sh_End ==
  In1 : Inport
  Demux : Demux  Outputs=3
  tag scope: Speed_M3=global, power_rota_M3=global, torque_M3=global
  wires:
  In1/1 -> Demux/1
  Demux/1 -> [power_rota_M3]
  Demux/2 -> [torque_M3]
  Demux/3 -> [Speed_M3]
